simulink model "soh_codegen"  (R2015b)
settings: Solver=FixedStepAuto  StartTime=0.0  StopTime=inf  FixedStep=sohk_stepSize  RelTol=1e-3  SampleTimeConstraint=STIndependent
undefined symbols (not defined in the file): bmsc_InternalChgResistX, bmsc_InternalChgResistY, bmsc_InternalChgResistZ, bmsc_InternalDischgResistX, bmsc_InternalDischgResistY, bmsc_InternalDischgResistZ, sohc_current_threshold, sohc_customer_filter_coeff, sohc_filter_coeff, sohc_pct_R_limit, sohk_CellBalancingResistor, sohk_delta_time, sohk_last_sohr, sohk_stepSize, sohv_factoryInit_sohc, sohv_factoryInit_sohr
libraries: simulink x1
settings Model: PauseTimes=22  Creator=favv5g  LastModifiedBy=nctzv8
settings ConfigSet: Description=OpenECU configuration set for code generation under RTW-EC.
settings SolverCC: PositivePriorityOrder=on
settings DataIOCC: SaveFormat=Array  SignalLoggingSaveFormat=ModelDataLogs
settings OptimizationCC: DefaultParameterBehavior=Inlined  InlineInvariantSignals=on  ExpressionDepthLimit=2147483647  StateBitsets=on  DataBitsets=on  ZeroExternalMemoryAtStartup=off  ZeroInternalMemoryAtStartup=off  NoFixptDivByZeroProtection=on  EfficientFloat2IntCast=on  OptimizeModelRefInitCode=on  LifeSpan=1
settings DebuggingCC: SaveWithParameterizedLinksMsg=none  UnderspecifiedInitializationDetection=Classic  MergeDetectMultiDrivingBlocksExec=none  SignalResolutionControl=TryResolveAllWithWarning  MultiTaskDSMMsg=warning  MultiTaskCondExecSysMsg=none  SingleTaskRateTransMsg=error  CheckMatrixSingularityMsg=warning  VectorMatrixConversionMsg=warning  FcnCallInpInsideContextMsg=UseLocalSettings  SignalLabelMismatchMsg=warning  StateNameClashWarn=warning
settings HardwareCC: ProdBitPerPointer=32  ProdLargestAtomicInteger=Long  ProdLargestAtomicFloat=Double  ProdEndianess=BigEndian  ProdWordSize=32  ProdHWDeviceType=Freescale->32-bit PowerPC  TargetIntDivRoundTo=Zero  TargetEndianess=BigEndian  TargetHWDeviceType=Freescale->32-bit PowerPC  ProdEqTarget=off
settings RTWCC: SystemTargetFile=openecu_ert.tlc  MakeCommand=make_rtw optimized_floating_point=1  TemplateMakefile=openecu_ert_r2015b_64.tmf  Description=OpenECU Platform Target (ERT, optimised floating-point code)  RetainRTWFile=on  IncludeHyperlinkInReport=on
settings CodeAppCC: ForceParamTrailComments=on  IgnoreCustomStorageClasses=off  SimulinkDataObjDesc=on  CustomSymbolStrType=$N$R$M  InsertBlockDesc=on  InternalIdentifier=Classic
settings STFCustomTargetCC: TargetLibSuffix=.a  GenerateSampleERTMain=on  ConcurrentExecutionCompliant=off  IncludeMdlTerminateFcn=off  GeneratePreprocessorConditionals=Use local settings  CombineOutputUpdateFcns=on  IncludeFileDelimiter=UseQuote  ERTCustomFileBanners=on  SupportContinuousTime=off  MATLABClassNameForMDSCustomization=Simulink.SoftwareTarget.ERTCustomization  CPPClassGenCompliant=off  GRTInterface=off  SystemTargetFile=openecu_ert.tlc
settings ERTTargetCC: GenerateSampleERTMain=on  ParMdlRefBuildCompliant=off  CompOptLevelCompliant=off  ConcurrentExecutionCompliant=off  IncludeMdlTerminateFcn=off  ERTFirstTimeCompliant=off  IncludeFileDelimiter=UseQuote  SupportNonInlinedSFcns=on  ModelStepFunctionPrototypeControlCompliant=off  CPPClassGenCompliant=off  UseToolchainInfoCompliant=off  ExtModeMexFile=noextcomm  InlinedParameterPlacement=NonHierarchical  ERTSrcFileBannerTemplate=oe_code_c_template.cgt  ERTHdrFileBannerTemplate=oe_code_h_template.cgt  ERTDataSrcFileTemplate=oe_data_c_template.cgt  ERTDataHdrFileTemplate=oe_data_h_template.cgt  ERTCustomFileTemplate=example_file_process.tlc  GlobalDataDefinition=InSeparateSourceFile  GlobalDataReference=InSeparateHeaderFile  EnableUserReplacementTypes=on

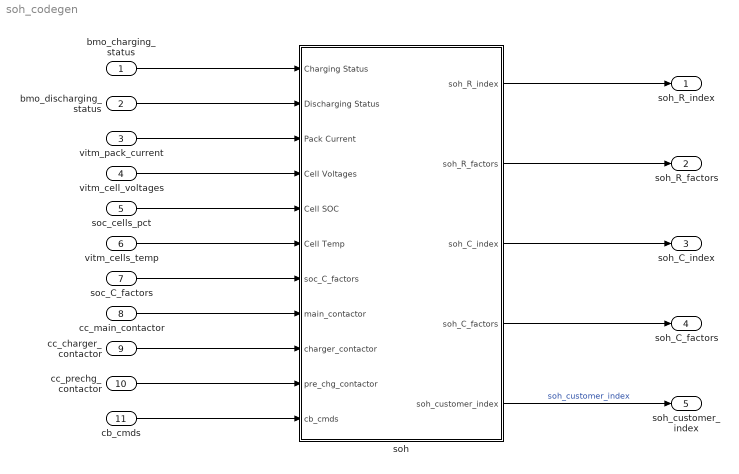
== system soh_codegen ==
  bmo_charging_status : Inport
  bmo_discharging_status : Inport  Port=2
  vitm_pack_current : Inport  Port=3
  vitm_cell_voltages : Inport  Port=4  PortDimensions=40
  soc_cells_pct : Inport  Port=5  PortDimensions=40
  vitm_cells_temp : Inport  Port=6  PortDimensions=40
  soc_C_factors : Inport  Port=7  PortDimensions=40
  cc_main_contactor : Inport  Port=8
  cc_charger_contactor : Inport  Port=9
  cc_prechg_contactor : Inport  Port=10
  cb_cmds : Inport  Port=11  OutDataTypeStr=boolean  PortDimensions=40
  soh : Subsystem  TreatAsAtomicUnit=on
  soh_R_index : Outport
  soh_R_factors : Outport  Port=2  PortDimensions=40
  soh_C_index : Outport  Port=3
  soh_C_factors : Outport  Port=4  PortDimensions=40  InitialOutput=sohv_factoryInit_sohc
  soh_customer_index : Outport  Port=5
  wires:
  bmo_charging_status/1 -> soh/1(Charging Status)
  bmo_discharging_status/1 -> soh/2(Discharging Status)
  vitm_pack_current/1 -> soh/3(Pack Current)
  vitm_cell_voltages/1 -> soh/4(Cell Voltages)
  soc_cells_pct/1 -> soh/5(Cell SOC)
  vitm_cells_temp/1 -> soh/6(Cell Temp)
  soh/1(soh_R_index) -> soh_R_index/1
  soc_C_factors/1 -> soh/7(soc_C_factors)
  soh/4(soh_C_factors) -> soh_C_factors/1
  soh/3(soh_C_index) -> soh_C_index/1
  soh/2(soh_R_factors) -> soh_R_factors/1
  soh/5(soh_customer_index) -> soh_customer_index/1  "soh_customer_index"
  cc_main_contactor/1 -> soh/8(main_contactor)
  cc_charger_contactor/1 -> soh/9(charger_contactor)
  cc_prechg_contactor/1 -> soh/10(pre_chg_contactor)
  cb_cmds/1 -> soh/11(cb_cmds)

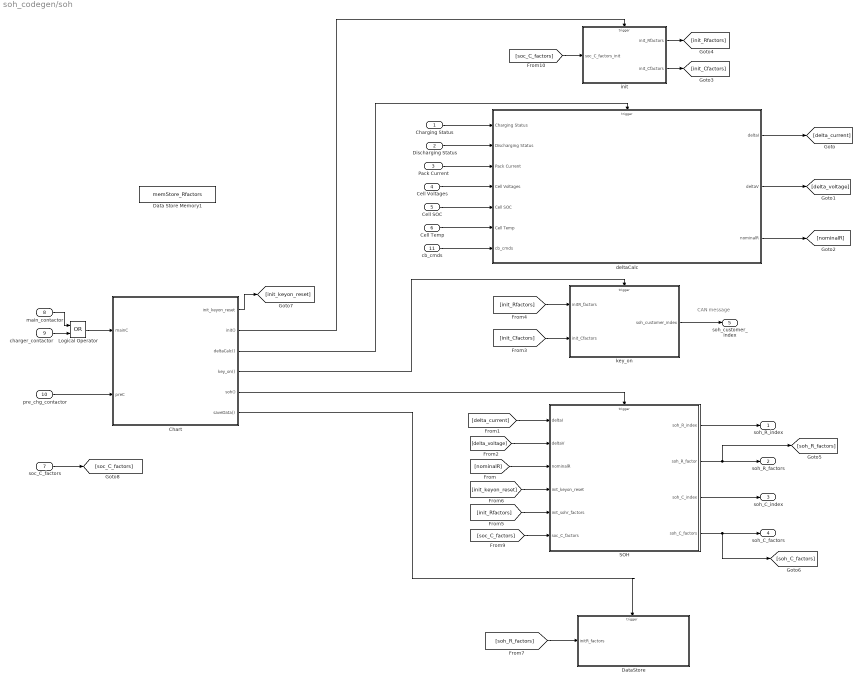
== system soh_codegen/soh ==
  note: CAN message
  Charging Status : Inport  OutDataTypeStr=boolean
  Discharging Status : Inport  Port=2  OutDataTypeStr=boolean
  Pack Current : Inport  Port=3
  Cell Voltages : Inport  Port=4  PortDimensions=40
  Cell SOC : Inport  Port=5  PortDimensions=40
  Cell Temp : Inport  Port=6  PortDimensions=40
  soc_C_factors : Inport  Port=7  PortDimensions=40
  main_contactor : Inport  Port=8
  charger_contactor : Inport  Port=9
  pre_chg_contactor : Inport  Port=10
  cb_cmds : Inport  Port=11  PortDimensions=40
  Chart : Stateflow chart  TreatAsAtomicUnit=on
  Data Store Memory1 : DataStoreMemory  DataStoreName=memStore_Rfactors  ReadBeforeWriteMsg=warning  WriteAfterWriteMsg=warning  WriteAfterReadMsg=warning  InitialValue=sohv_factoryInit_sohr
  DataStore : Subsystem
  Logical Operator : Logic  Operator=OR  AllPortsSameDT=off  OutDataTypeStr=boolean
  SOH : Subsystem
  deltaCalc : Subsystem
  init : Subsystem
  key_on : Subsystem
  soh_R_index : Outport
  soh_R_factors : Outport  Port=2
  soh_C_index : Outport  Port=3
  soh_C_factors : Outport  Port=4  PortDimensions=40
  soh_customer_index : Outport  Port=5
  wires:
  Charging Status/1 -> deltaCalc/1(Charging Status)
  Discharging Status/1 -> deltaCalc/2(Discharging Status)
  Pack Current/1 -> deltaCalc/3(Pack Current)
  Cell Voltages/1 -> deltaCalc/4(Cell Voltages)
  Cell SOC/1 -> deltaCalc/5(Cell SOC)
  Cell Temp/1 -> deltaCalc/6(Cell Temp)
  deltaCalc/3(nominalR) -> [nominalR]
  SOH/1(soh_R_index) -> soh_R_index/1
  SOH/2(soh_R_factor) -> [soh_R_factors], soh_R_factors/1
  [delta_voltage] -> SOH/2(deltaV)
  [delta_current] -> SOH/1(deltaI)
  [nominalR] -> SOH/3(nominalR)
  init/2(init_Cfactors) -> [init_Cfactors]
  init/1(init_Rfactors) -> [init_Rfactors]
  SOH/3(soh_C_index) -> soh_C_index/1
  SOH/4(soh_C_factors) -> [soh_C_factors], soh_C_factors/1
  key_on/1(soh_customer_index) -> soh_customer_index/1
  [init_Cfactors] -> key_on/2(init_Cfactors)
  [init_Rfactors] -> key_on/1(initR_factors)
  [init_Rfactors] -> SOH/5(init_sohr_factors)
  [init_keyon_reset] -> SOH/4(init_keyon_reset)
  Chart/1(init_keyon_reset) -> [init_keyon_reset]
  Chart/2(init()) -> init/Trigger
  Chart/3(deltaCalc()) -> deltaCalc/Trigger
  Chart/4(key_on()) -> key_on/Trigger
  Chart/5(soh()) -> SOH/Trigger
  Chart/6(saveData()) -> DataStore/Trigger
  pre_chg_contactor/1 -> Chart/2(preC)
  main_contactor/1 -> Logical Operator/1
  charger_contactor/1 -> Logical Operator/2
  Logical Operator/1 -> Chart/1(mainC)
  [soh_R_factors] -> DataStore/1(initR_factors)
  soc_C_factors/1 -> [soc_C_factors]
  [soc_C_factors] -> SOH/6(soc_C_factors)
  [soc_C_factors] -> init/1(soc_C_factors_init)
  cb_cmds/1 -> deltaCalc/7(cb_cmds)
  deltaCalc/1(deltaI) -> [delta_current]
  deltaCalc/2(deltaV) -> [delta_voltage]

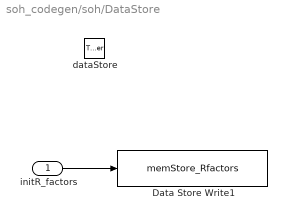
== system soh_codegen/soh/DataStore ==
  initR_factors : Inport
  dataStore : TriggerPort  TriggerType=function-call  PortDimensions=1
  Data Store Write1 : DataStoreWrite  DataStoreName=memStore_Rfactors
  wires:
  initR_factors/1 -> Data Store Write1/1

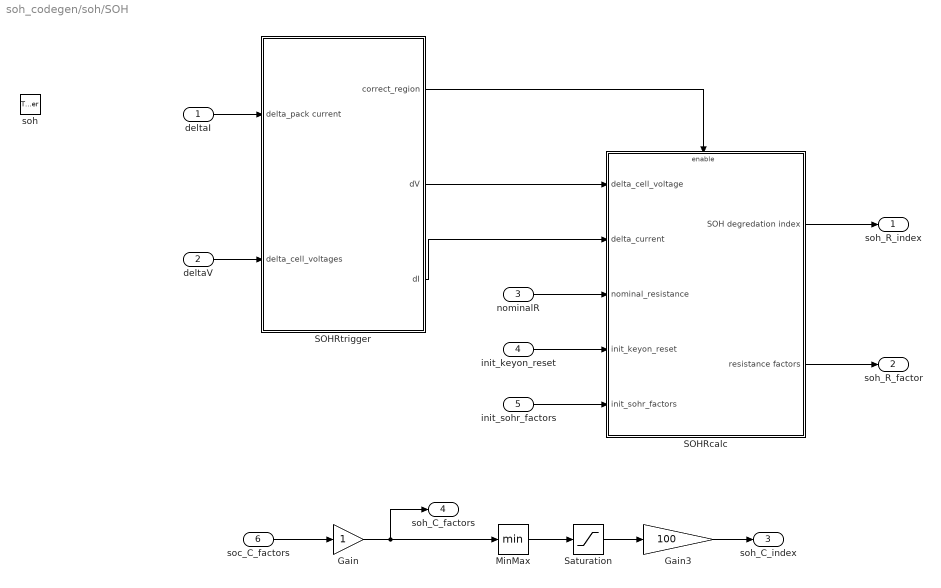
== system soh_codegen/soh/SOH ==
  deltaI : Inport
  deltaV : Inport  Port=2
  nominalR : Inport  Port=3
  init_keyon_reset : Inport  Port=4
  init_sohr_factors : Inport  Port=5  PortDimensions=40
  soc_C_factors : Inport  Port=6  PortDimensions=40
  soh : TriggerPort  TriggerType=function-call  PortDimensions=1
  Gain : Gain
  Gain3 : Gain  Gain=100
  MinMax : MinMax
  SOHRcalc : Subsystem
  SOHRtrigger : Subsystem
  Saturation : Saturate  UpperLimit=1  LowerLimit=0
  soh_R_index : Outport
  soh_R_factor : Outport  Port=2
  soh_C_index : Outport  Port=3
  soh_C_factors : Outport  Port=4  PortDimensions=40
  wires:
  nominalR/1 -> SOHRcalc/3(nominal_resistance)
  deltaI/1 -> SOHRtrigger/1(delta_pack current)
  SOHRtrigger/3(dI) -> SOHRcalc/2(delta_current)
  SOHRcalc/2(" resistance factors") -> soh_R_factor/1
  SOHRtrigger/2(dV) -> SOHRcalc/1(delta_cell_voltage)
  SOHRtrigger/1(correct_region) -> SOHRcalc/Enable
  SOHRcalc/1(SOH degredation index) -> soh_R_index/1
  deltaV/1 -> SOHRtrigger/2(delta_cell_voltages)
  soc_C_factors/1 -> Gain/1
  Gain/1 -> soh_C_factors/1, MinMax/1
  Saturation/1 -> Gain3/1
  MinMax/1 -> Saturation/1
  Gain3/1 -> soh_C_index/1
  init_sohr_factors/1 -> SOHRcalc/5(init_sohr_factors)
  init_keyon_reset/1 -> SOHRcalc/4(init_keyon_reset)

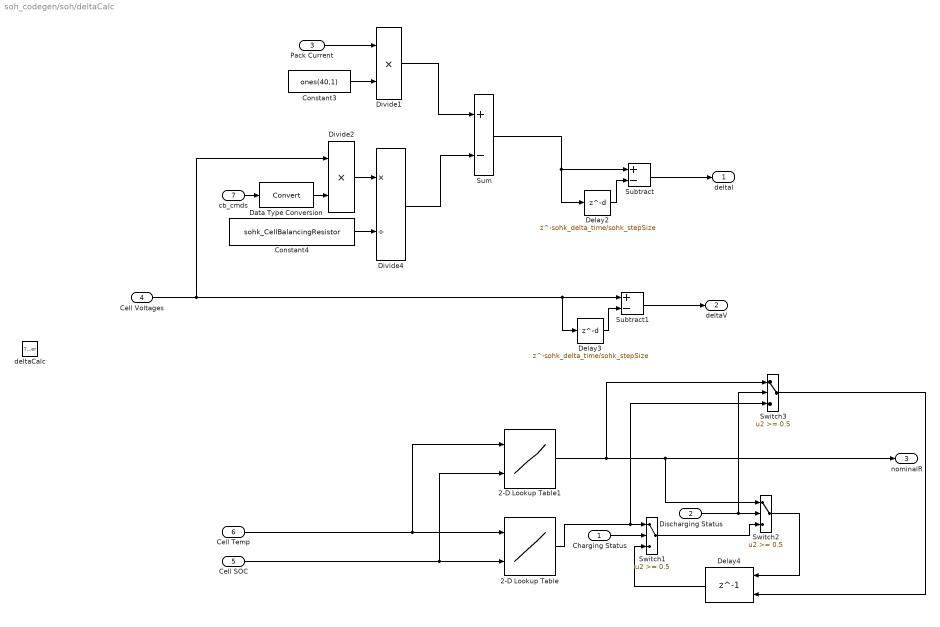
== system soh_codegen/soh/deltaCalc ==
  Charging Status : Inport  OutDataTypeStr=boolean
  Discharging Status : Inport  Port=2  OutDataTypeStr=boolean
  Pack Current : Inport  Port=3
  Cell Voltages : Inport  Port=4  PortDimensions=40
  Cell SOC : Inport  Port=5  PortDimensions=40
  Cell Temp : Inport  Port=6  PortDimensions=40
  cb_cmds : Inport  Port=7
  deltaCalc : TriggerPort  TriggerType=function-call  PortDimensions=1
  2-D Lookup Table : Lookup_n-D  BreakpointsForDimension1=bmsc_InternalChgResistX  BreakpointsForDimension2=bmsc_InternalChgResistY  Table=bmsc_InternalChgResistZ  InternalRulePriority=Speed  RndMeth=Simplest  InputSameDT=on
  2-D Lookup Table1 : Lookup_n-D  BreakpointsForDimension1=bmsc_InternalDischgResistX  BreakpointsForDimension2=bmsc_InternalDischgResistY  Table=bmsc_InternalDischgResistZ  InternalRulePriority=Speed  RndMeth=Simplest  InputSameDT=on
  Constant3 : Constant  Value=ones(40,1)
  Constant4 : Constant  Value=sohk_CellBalancingResistor
  Data Type Conversion : DataTypeConversion
  Delay2 : Delay  DelayLength=sohk_delta_time/sohk_stepSize
  Delay3 : Delay  DelayLength=sohk_delta_time/sohk_stepSize
  Delay4 : Delay  DelayLength=1  InitialConditionSource=Input port
      settings: InputPortMap=u0,p4
  Divide1 : Product  Inputs=**
  Divide2 : Product  Inputs=**
  Divide4 : Product  Inputs=*/
  Subtract : Sum  Inputs=+-
  Subtract1 : Sum  Inputs=+-
  Sum : Sum  Inputs=+-
  Switch1 : Switch  Threshold=0.5
  Switch2 : Switch  Threshold=0.5
  Switch3 : Switch  Threshold=0.5
  deltaI : Outport
  deltaV : Outport  Port=2
  nominalR : Outport  Port=3
  wires:
  Subtract/1 -> deltaI/1
  Delay3/1 -> Subtract1/2
  Charging Status/1 -> Switch1/2
  Delay4/1 -> Switch1/3
  Cell SOC/1 -> 2-D Lookup Table1/2, 2-D Lookup Table/2
  Switch2/1 -> Delay4/1
  Subtract1/1 -> deltaV/1
  Delay2/1 -> Subtract/2
  Cell Temp/1 -> 2-D Lookup Table1/1, 2-D Lookup Table/1
  2-D Lookup Table/1 -> Switch3/3, Switch1/1
  Pack Current/1 -> Divide1/1
  Constant3/1 -> Divide1/2
  Cell Voltages/1 -> Divide2/1, Delay3/1, Subtract1/1
  cb_cmds/1 -> Data Type Conversion/1
  Divide2/1 -> Divide4/1
  Constant4/1 -> Divide4/2
  Divide1/1 -> Sum/1
  Divide4/1 -> Sum/2
  Data Type Conversion/1 -> Divide2/2
  Sum/1 -> Delay2/1, Subtract/1
  2-D Lookup Table1/1 -> nominalR/1, Switch2/1, Switch3/1
  Discharging Status/1 -> Switch3/2, Switch2/2
  Switch1/1 -> Switch2/3
  Switch3/1 -> Delay4/2

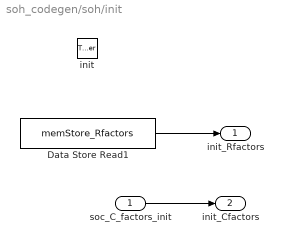
== system soh_codegen/soh/init ==
  soc_C_factors_init : Inport
  init : TriggerPort  TriggerType=function-call  PortDimensions=1
  Data Store Read1 : DataStoreRead  DataStoreName=memStore_Rfactors
  init_Rfactors : Outport
  init_Cfactors : Outport  Port=2
  wires:
  soc_C_factors_init/1 -> init_Cfactors/1
  Data Store Read1/1 -> init_Rfactors/1

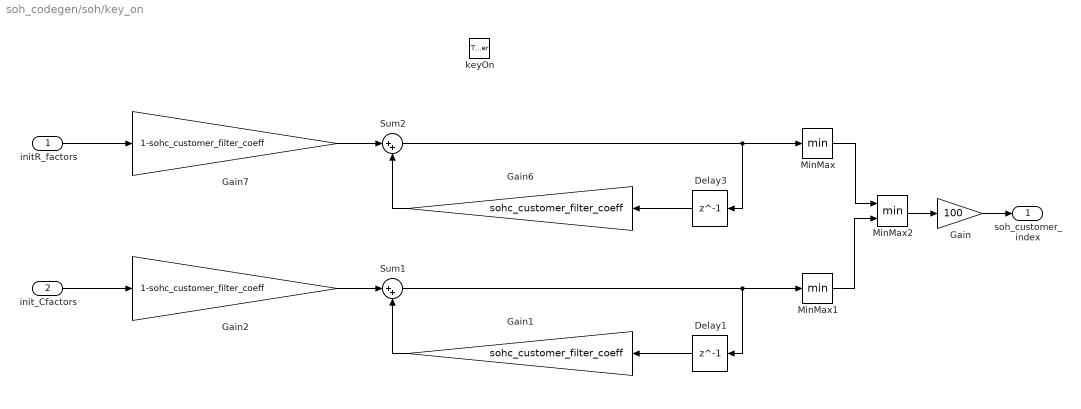
== system soh_codegen/soh/key_on ==
  initR_factors : Inport
  init_Cfactors : Inport  Port=2
  keyOn : TriggerPort  TriggerType=function-call  PortDimensions=1
  Delay1 : Delay  DelayLength=1  InitialCondition=sohv_factoryInit_sohc
  Delay3 : Delay  DelayLength=1  InitialCondition=sohv_factoryInit_sohr
  Gain : Gain  Gain=100
  Gain1 : Gain  Gain=sohc_customer_filter_coeff
  Gain2 : Gain  Gain=1-sohc_customer_filter_coeff
  Gain6 : Gain  Gain=sohc_customer_filter_coeff
  Gain7 : Gain  Gain=1-sohc_customer_filter_coeff
  MinMax : MinMax
  MinMax1 : MinMax
  MinMax2 : MinMax  Inputs=2
  Sum1 : Sum  Inputs=|++
  Sum2 : Sum  Inputs=|++
  soh_customer_index : Outport
  wires:
  MinMax1/1 -> MinMax2/2
  MinMax/1 -> MinMax2/1
  Delay1/1 -> Gain1/1
  Gain1/1 -> Sum1/2
  Sum1/1 -> MinMax1/1, Delay1/1
  Gain2/1 -> Sum1/1
  Delay3/1 -> Gain6/1
  Sum2/1 -> MinMax/1, Delay3/1
  Gain6/1 -> Sum2/2
  Gain7/1 -> Sum2/1
  initR_factors/1 -> Gain7/1
  init_Cfactors/1 -> Gain2/1
  MinMax2/1 -> Gain/1
  Gain/1 -> soh_customer_index/1

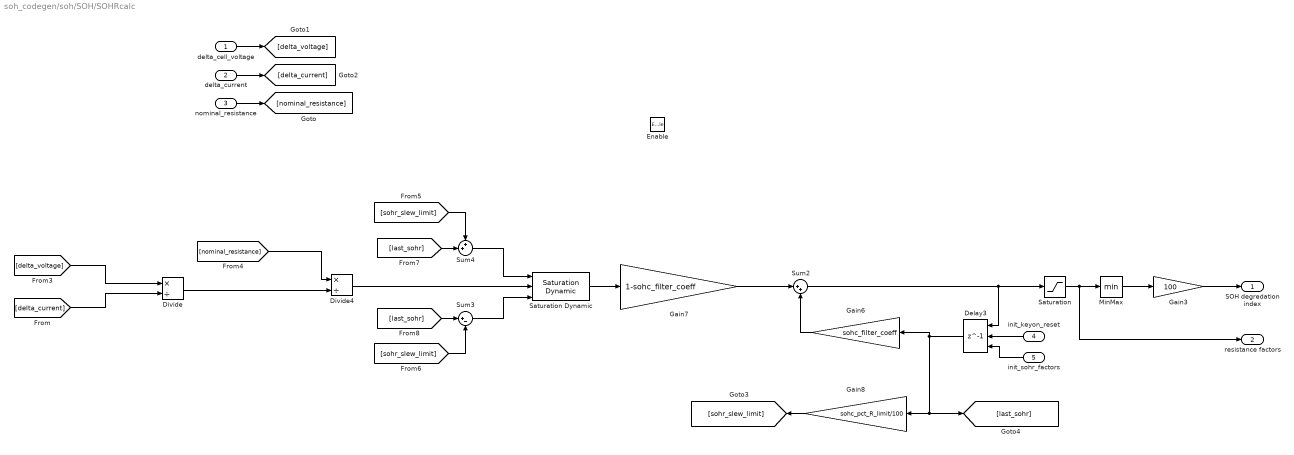
== system soh_codegen/soh/SOH/SOHRcalc ==
  delta_cell_voltage : Inport
  delta_current : Inport  Port=2
  nominal_resistance : Inport  Port=3
  init_keyon_reset : Inport  Port=4
  init_sohr_factors : Inport  Port=5
  Enable : EnablePort
  Delay3 : Delay  DelayLength=1  InitialConditionSource=Input port  InitialCondition=sohk_last_sohr  ExternalReset=Rising
      settings: InputPortMap=u0,r5,p4
  Divide : Product  Inputs=*/
  Divide4 : Product  Inputs=*/
  Gain3 : Gain  Gain=100
  Gain6 : Gain  Gain=sohc_filter_coeff
  Gain7 : Gain  Gain=1-sohc_filter_coeff
  Gain8 : Gain  Gain=sohc_pct_R_limit/100
  MinMax : MinMax
  Saturation : Saturate  UpperLimit=1  LowerLimit=0
  Saturation Dynamic : simulink/Discontinuities/Saturation Dynamic  OutMin=[]  OutMax=[]  OutDataTypeStr=Inherit: Same as second input  OutDataType=fixdt(1, 16)  OutScaling=2^-10  DoSatur=off
  Sum2 : Sum  Inputs=|++
  Sum3 : Sum  Inputs=|+-
  Sum4 : Sum  Inputs=++|
  SOH degredation index : Outport
  " resistance factors" : Outport  Port=2
  wires:
  [delta_voltage] -> Divide/1
  [delta_current] -> Divide/2
  nominal_resistance/1 -> [nominal_resistance]
  delta_cell_voltage/1 -> [delta_voltage]
  delta_current/1 -> [delta_current]
  Divide/1 -> Divide4/2
  [nominal_resistance] -> Divide4/1
  Divide4/1 -> Saturation Dynamic/2
  Delay3/1 -> Gain6/1, [last_sohr], Gain8/1
  Gain6/1 -> Sum2/2
  Gain7/1 -> Sum2/1
  Saturation Dynamic/1 -> Gain7/1
  MinMax/1 -> Gain3/1
  Sum2/1 -> Delay3/1, Saturation/1
  Saturation/1 -> " resistance factors"/1, MinMax/1
  Gain3/1 -> SOH degredation index/1
  Gain8/1 -> [sohr_slew_limit]
  Sum4/1 -> Saturation Dynamic/1
  [sohr_slew_limit] -> Sum4/1
  [sohr_slew_limit] -> Sum3/2
  [last_sohr] -> Sum4/2
  [last_sohr] -> Sum3/1
  Sum3/1 -> Saturation Dynamic/3
  init_keyon_reset/1 -> Delay3/2
  init_sohr_factors/1 -> Delay3/3

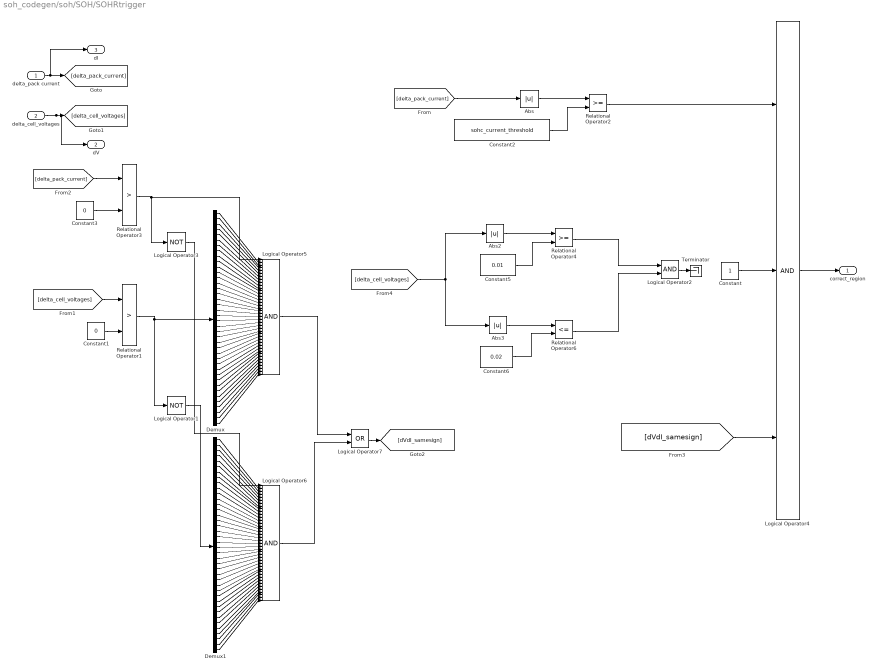
== system soh_codegen/soh/SOH/SOHRtrigger ==
  delta_pack current : Inport
  delta_cell_voltages : Inport  Port=2
  Abs : Abs
  Abs2 : Abs
  Abs3 : Abs
  Constant : Constant
  Constant1 : Constant  Value=0
  Constant2 : Constant  Value=sohc_current_threshold
  Constant3 : Constant  Value=0
  Constant5 : Constant  Value=0.01
  Constant6 : Constant  Value=0.02
  Demux : Demux  Outputs=40
  Demux1 : Demux  Outputs=40
  Logical Operator1 : Logic  Operator=NOT  AllPortsSameDT=off  OutDataTypeStr=boolean
  Logical Operator2 : Logic  AllPortsSameDT=off  OutDataTypeStr=boolean
  Logical Operator3 : Logic  Operator=NOT  AllPortsSameDT=off  OutDataTypeStr=boolean
  Logical Operator4 : Logic  Inputs=3  AllPortsSameDT=off  OutDataTypeStr=boolean
  Logical Operator5 : Logic  Inputs=41  AllPortsSameDT=off  OutDataTypeStr=boolean
  Logical Operator6 : Logic  Inputs=41  AllPortsSameDT=off  OutDataTypeStr=boolean
  Logical Operator7 : Logic  Operator=OR  AllPortsSameDT=off  OutDataTypeStr=boolean
  Relational Operator1 : RelationalOperator  Operator=>  OutDataTypeStr=boolean
  Relational Operator2 : RelationalOperator  OutDataTypeStr=boolean
  Relational Operator3 : RelationalOperator  Operator=>  OutDataTypeStr=boolean
  Relational Operator4 : RelationalOperator  OutDataTypeStr=boolean
  Relational Operator6 : RelationalOperator  Operator=<=  OutDataTypeStr=boolean
  Terminator : Terminator
  correct_region : Outport
  dV : Outport  Port=2
  dI : Outport  Port=3
  wires:
  Abs/1 -> Relational Operator2/1
  Constant2/1 -> Relational Operator2/2
  Logical Operator4/1 -> correct_region/1
  delta_pack current/1 -> dI/1, [delta_pack_current]
  [delta_pack_current] -> Abs/1
  delta_cell_voltages/1 -> dV/1, [delta_cell_voltages]
  [delta_cell_voltages] -> Relational Operator1/1
  Constant1/1 -> Relational Operator1/2
  [delta_pack_current] -> Relational Operator3/1
  Constant3/1 -> Relational Operator3/2
  Abs2/1 -> Relational Operator4/1
  Constant5/1 -> Relational Operator4/2
  Abs3/1 -> Relational Operator6/1
  Constant6/1 -> Relational Operator6/2
  [delta_cell_voltages] -> Abs3/1, Abs2/1
  Relational Operator2/1 -> Logical Operator4/1
  Relational Operator4/1 -> Logical Operator2/1
  Relational Operator6/1 -> Logical Operator2/2
  Constant/1 -> Logical Operator4/2
  [dVdI_samesign] -> Logical Operator4/3
  Relational Operator1/1 -> Demux/1, Logical Operator1/1
  Relational Operator3/1 -> Logical Operator5/1, Logical Operator3/1
  Demux/1 -> Logical Operator5/2
  Demux/2 -> Logical Operator5/3
  Demux/3 -> Logical Operator5/4
  Demux/4 -> Logical Operator5/5
  Demux/5 -> Logical Operator5/6
  Demux/6 -> Logical Operator5/7
  Demux/7 -> Logical Operator5/8
  Demux/8 -> Logical Operator5/9
  Demux/9 -> Logical Operator5/10
  Demux/10 -> Logical Operator5/11
  Demux/11 -> Logical Operator5/12
  Demux/12 -> Logical Operator5/13
  Demux/13 -> Logical Operator5/14
  Demux/14 -> Logical Operator5/15
  Demux/15 -> Logical Operator5/16
  Demux/16 -> Logical Operator5/17
  Demux/17 -> Logical Operator5/18
  Demux/18 -> Logical Operator5/19
  Demux/19 -> Logical Operator5/20
  Demux/20 -> Logical Operator5/21
  Demux/21 -> Logical Operator5/22
  Demux/22 -> Logical Operator5/23
  Demux/23 -> Logical Operator5/24
  Demux/24 -> Logical Operator5/25
  Demux/25 -> Logical Operator5/26
  Demux/26 -> Logical Operator5/27
  Demux/27 -> Logical Operator5/28
  Demux/28 -> Logical Operator5/29
  Demux/29 -> Logical Operator5/30
  Demux/30 -> Logical Operator5/31
  Demux/31 -> Logical Operator5/32
  Demux/32 -> Logical Operator5/33
  Demux/33 -> Logical Operator5/34
  Demux/34 -> Logical Operator5/35
  Demux/35 -> Logical Operator5/36
  Demux/36 -> Logical Operator5/37
  Demux/37 -> Logical Operator5/38
  Demux/38 -> Logical Operator5/39
  Demux/39 -> Logical Operator5/40
  Demux/40 -> Logical Operator5/41
  Logical Operator1/1 -> Demux1/1
  Demux1/1 -> Logical Operator6/2
  Demux1/2 -> Logical Operator6/3
  Demux1/3 -> Logical Operator6/4
  Demux1/4 -> Logical Operator6/5
  Demux1/5 -> Logical Operator6/6
  Demux1/6 -> Logical Operator6/7
  Demux1/7 -> Logical Operator6/8
  Demux1/8 -> Logical Operator6/9
  Demux1/9 -> Logical Operator6/10
  Demux1/10 -> Logical Operator6/11
  Demux1/11 -> Logical Operator6/12
  Demux1/12 -> Logical Operator6/13
  Demux1/13 -> Logical Operator6/14
  Demux1/14 -> Logical Operator6/15
  Demux1/15 -> Logical Operator6/16
  Demux1/16 -> Logical Operator6/17
  Demux1/17 -> Logical Operator6/18
  Demux1/18 -> Logical Operator6/19
  Demux1/19 -> Logical Operator6/20
  Demux1/20 -> Logical Operator6/21
  Demux1/21 -> Logical Operator6/22
  Demux1/22 -> Logical Operator6/23
  Demux1/23 -> Logical Operator6/24
  Demux1/24 -> Logical Operator6/25
  Demux1/25 -> Logical Operator6/26
  Demux1/26 -> Logical Operator6/27
  Demux1/27 -> Logical Operator6/28
  Demux1/28 -> Logical Operator6/29
  Demux1/29 -> Logical Operator6/30
  Demux1/30 -> Logical Operator6/31
  Demux1/31 -> Logical Operator6/32
  Demux1/32 -> Logical Operator6/33
  Demux1/33 -> Logical Operator6/34
  Demux1/34 -> Logical Operator6/35
  Demux1/35 -> Logical Operator6/36
  Demux1/36 -> Logical Operator6/37
  Demux1/37 -> Logical Operator6/38
  Demux1/38 -> Logical Operator6/39
  Demux1/39 -> Logical Operator6/40
  Demux1/40 -> Logical Operator6/41
  Logical Operator3/1 -> Logical Operator6/1
  Logical Operator5/1 -> Logical Operator7/1
  Logical Operator6/1 -> Logical Operator7/2
  Logical Operator7/1 -> [dVdI_samesign]
  Logical Operator2/1 -> Terminator/1

== stateflow chart soh_codegen/soh/Chart ==
  state key_ON
    entry:
    init_keyon_reset = 1;
    (default) -> (junction 66)
    key_ON -> (junction 66) [order 1]
    (junction 66) -> (junction 3) : {init;}
    (junction 3) -> (junction 5) : {key_on;}
    (junction 5) -> (junction 37) : {deltaCalc;}
    (junction 37) -> (junction 61) : {soh;}
  state sohr
    entry:
    init_keyon_reset = 0;
    (default) -> (junction 18)
    sohr -> (junction 18) [order 1]
    (junction 18) -> (junction 21) : {deltaCalc;}
    (junction 21) -> (junction 39) : {soh;}
  state dataStore
    entry:
    init_keyon_reset = 0;
    (default) -> (junction 47)
    dataStore -> (junction 47) [order 1]
    (junction 47) -> (junction 45) : {saveData;}
  state end
    entry:
  (default) -> key_ON
  end -> key_ON : [preC == 1 || mainC ==1]
  key_ON -> sohr [order 1] : [preC == 1 || mainC == 1 ]
  sohr -> dataStore [order 1] : [mainC == 0 && preC == 0]
  dataStore -> end [order 1]
  data: mainC input boolean; preC input boolean; init_keyon_reset output
  events: init output FUNCTION_CALL_EVENT; deltaCalc output FUNCTION_CALL_EVENT; key_on output FUNCTION_CALL_EVENT; soh output FUNCTION_CALL_EVENT; saveData output FUNCTION_CALL_EVENT
